simulink model "cruise_control"  (Simulink 7.8)
settings: Solver=FixedStepDiscrete  SolverMode=SingleTasking  StartTime=0.0  StopTime=50  FixedStep=0.01  RelTol=1e-3  AbsTol=1e-6
model workspace (MAT data in the model file):
  converter_data = [0  137.465208994  2.232; 0.1  137.065019157  2.075; 0.2  135.864449646  1.975; 0.3  135.664354728  1.846; 0.4  137.565256453  1.72; 0.5  140.366585312  1.564; 0.6  145.268910814  1.409; 0.7  152.872517717  1.254; 0.8  162.9773111  1.096; 0.81  164.27792807  1.08; 0.82  166.178829795  1.061; 0.83  167.979684062  1.043; 0.84  170.080680706  1.028; 0.85  172.781962105  1.012; 0.86  175.383196045  1.002; 0.87  179.585189333  1.002; 0.88  183.587087703  1.001; 0.89  189.890077635  0.998; 0.9  197.693779455  0.999; 0.92  215.902417037  1.001; 0.94  244.515990379  1.002]
  emap = [-40  -44  -49  -53  -57  -61  -65  -70  -74  -78  -82; 215  117  85  66  44  29  10  -2  -13  -22  -32; 245  208  178  148  122  104  85  66  48  33  18; 264  260  241  219  193  167  152  133  119  96  85; 264  279  282  275  260  238  223  208  189  171  152; 267  290  293  297  290  275  260  256  234  212  193; 267  297  305  305  305  301  293  282  267  249  226; 267  301  308  312  319  323  319  316  297  279  253; 267  301  312  319  327  327  327  327  312  293  267; 267  301  312  319  327  334  334  334  319  305  275]
  Iei = 0.0219914882836
  nevec = [800 1200 1600 2000 2400 2800 3200 3600 4000 4400 4800]
  p0 = 0.07934
  p1 = 0.07934
  thvec = [0; 20; 30; 40; 50; 60; 70; 80; 90; 100]
  vehicledata : num (value not decoded)
values from neighbouring files (symbols this model uses):
  cruise_ki = 0.01    [cruise_control_data.m]    (also in fxpdata_simulinkpackage.mat)
  cruise_kp = 0.02    [cruise_control_data.m]    (also in fxpdata_simulinkpackage.mat)
  target_max = 100    [cruise_control_data.m]    (also in fxpdata_simulinkpackage.mat)
  target_min = 30    [cruise_control_data.m]    (also in fxpdata_simulinkpackage.mat)
  throt_max = 100    [cruise_control_data.m]    (also in fxpdata_simulinkpackage.mat)
  throt_min = 0    [cruise_control_data.m]    (also in fxpdata_simulinkpackage.mat)
  vel_dec = 1    [cruise_control_data.m]    (also in fxpdata_simulinkpackage.mat)
  vel_inc = 1    [cruise_control_data.m]    (also in fxpdata_simulinkpackage.mat)
undefined symbols (not defined in the file or in its folder): DiscIntNeverNeededParam
libraries: simulink x1
Description:
  | ƒNƒ‹?[ƒYƒRƒ“ƒgƒ??[ƒ‹ƒ‚ƒfƒ‹
settings Model: MinMaxOverflowLogging=MinMaxAndOverflow  Creator=The MathWorks Inc.  LastModifiedBy=itoy  CovSaveName=covdata_cc  CovMetricSettings=dcmtr  CovHTMLOptions=-aTS=1 -bRG=1 -bTC=1 -hTR=0 -nFC=0 -scm=1 -bcm=1 -xEv=0  ExtModeTrigMode=oneshot  ExtModeArmWhenConnect=off  ExtModeAutoUpdateStatusClock=off
settings DataIOCC: LimitDataPoints=off  SaveFormat=StructureWithTime  SaveOutput=off  SignalLogging=off  DSMLogging=off  SaveTime=off  SignalLoggingName=mysig
settings OptimizationCC: InlineParams=on  UseIntDivNetSlope=on  InlineInvariantSignals=on  EnhancedBackFolding=on  EfficientFloat2IntCast=on  OptimizeModelRefInitCode=on  LifeSpan=1
settings DebuggingCC: SignalInfNanChecking=error  SaveWithParameterizedLinksMsg=none  CheckExecutionContextPreStartOutputMsg=on  CheckExecutionContextRuntimeOutputMsg=on  SolverPrmCheckMsg=none  SingleTaskRateTransMsg=error  IntegerOverflowMsg=error  UniqueDataStoreMsg=error  BusObjectLabelMismatch=error  RootOutportRequireBusObject=error  AssertControl=DisableAll  StrictBusMsg=ErrorOnBusTreatedAsVector  BusNameAdapt=ErrorWithoutRepair  NonBusSignalsTreatedAsBus=error  LoggingUnavailableSignals=none
settings HardwareCC: ProdIntDivRoundTo=Zero  ProdEndianess=LittleEndian  ProdHWDeviceType=NEC->V850  TargetIntDivRoundTo=Zero  TargetEndianess=LittleEndian  TargetHWDeviceType=MATLAB Host
settings ModelReferenceCC: ModelReferenceNumInstancesAllowed=Single
settings SFSimCC: SFSimEcho=off  SimParseCustomCode=off
settings RTWCC: SystemTargetFile=ert.tlc  TemplateMakefile=ert_default_tmf  Description=Real-Time Workshop Embedded Coder  GenerateReport=on  ProcessScript=ert_make_rtw_hook  IncludeHyperlinkInReport=on  LaunchReport=on  IncludeERTFirstTime=on  RTWCompilerOptimization=On
settings CodeAppCC: IgnoreCustomStorageClasses=off
settings ERTTargetCC: MultiwordLength=2048  GenerateSampleERTMain=on  GenerateErtSFunction=on  CreateSILPILBlock=SIL  InlinedParameterPlacement=NonHierarchical  ERTCustomFileTemplate=example_file_process.tlc  ConvertIfToSwitch=off  SuppressUnreachableDefaultCases=off
settings ConfigComp: Description=Design Verifier Custom Configuration Component  DVMaxProcessTime=3000  DVDisplayUnsatisfiableObjectives=on  DVModelCoverageObjectives=MCDC  DVMaxTestCaseSteps=500  DVTestSuiteOptimization=CombinedObjectives  DVSaveReport=on

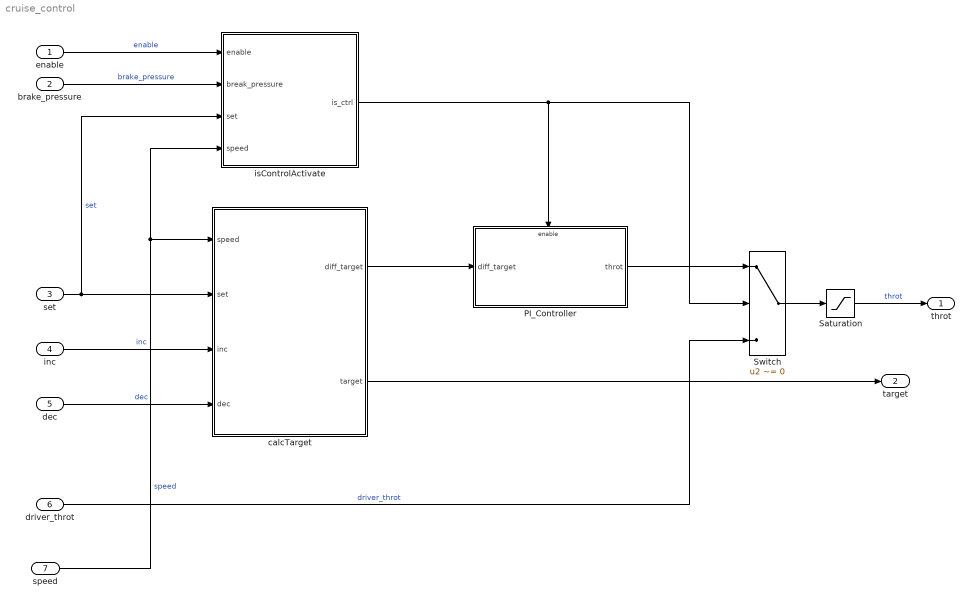
== system cruise_control ==
  enable : Inport  PortDimensions=1  Interpolate=off
  brake_pressure : Inport  Port=2  PortDimensions=1  Interpolate=off
  set : Inport  Port=3  PortDimensions=1  Interpolate=off
  inc : Inport  Port=4  PortDimensions=1  Interpolate=off
  dec : Inport  Port=5  PortDimensions=1  Interpolate=off
  driver_throt : Inport  Port=6  PortDimensions=1  Interpolate=off
  speed : Inport  Port=7  PortDimensions=1  Interpolate=off
  PI_Controller : Subsystem  RequirementInfo={'other' 'cruisecontrol_spec.xls' '@Simulink_requirement_item_13' 'true' 'ƒXƒ?ƒbƒgƒ‹ŒvŽZ' '' ; 'other' 'cruisecontrol_spec.xls' '@Simulink_requirement_item_14' 'true' 'ƒXƒ?ƒbƒgƒ‹’l‚Í?API?§Œä‚É‚æ‚èŒvŽZ‚³‚ê‚é?B' '' } %GIDa_c9cd3625_12f4_4b7c_a41d_1cb041b9c58f
  Saturation : Saturate  RequirementInfo={'other' 'cruisecontrol_spec.xls' '@Simulink_requirement_item_15' 'true' '?o—ÍƒXƒ?ƒbƒgƒ‹’l‚Í?Å‘åƒXƒ?ƒbƒgƒ‹’lˆÈ‰º?A?Å?¬ƒXƒ?ƒbƒgƒ‹’lˆÈ?ã‚Å‚ ‚é?B' '' } %GIDa_29e6bb04_5d3c_40ee_9701_e63e8e51ec96  UpperLimit=throt_max  LowerLimit=throt_min  OutDataTypeStr=Inherit: Inherit via back propagation
      settings: AttributesFormatString=<UpperLimit = %<UpperLimit>>\n<LowerLimit = %<LowerLimit>>
  Switch : Switch  RequirementInfo={'other' 'cruisecontrol_spec.xls' '@Simulink_requirement_item_16' 'true' '?§Œä‹–‰Â‚ªOFF‚Ì?Û‚É‚Í?Aƒhƒ‰ƒCƒo?[ƒXƒ?ƒbƒgƒ‹’l‚ªƒXƒ?ƒbƒgƒ‹’l‚Æ‚µ‚Ä?o—Í‚³‚ê‚é?B' '' } %GIDa_0f4dbb7e_1328_499c_8665_60d1af7bcbda  Criteria=u2 ~= 0  OutDataTypeStr=Inherit: Inherit via back propagation
      settings: AttributesFormatString=<Criteria=%<Criteria>>
  calcTarget : Subsystem  RequirementInfo={'other' 'cruisecontrol_spec.xls' '@Simulink_requirement_item_4' 'true' '–Ú•WŽÔ‘¬?Ý’è' '' } %GIDa_af1ad8a6_b9b3_46e5_9fb4_ba2528b86dbf
  isControlActivate : Subsystem  RequirementInfo={'other' 'cruisecontrol_spec.xls' '@Simulink_requirement_item_1' 'true' 'ƒNƒ‹?[ƒYƒRƒ“ƒgƒ??[ƒ‹—LŒø‰»”»’f' '' ; 'other' 'cruisecontrol_spec.xls' '@Simulink_requirement_item_2' 'true' '?§Œä‹–‰Â‚ÍŽŸ‚Ì?ðŒ?‚ª‘S‚Ä–ž‚½‚³‚ê‚é?ê?‡‚ÉON‚Æ‚È‚é?B ?E—LŒøƒXƒCƒbƒ`‚ªON ?EƒuƒŒ?[ƒL‚ªOFF ?EƒZƒbƒgƒXƒCƒbƒ`‚ªON‚à‚µ‚­‚Í?§Œä‹–‰Â‚Ì‘O‰ñ’l‚ªON ?EŽÔ‘¬‚ª–Ú•W?Å‘åˆÈ‰º‚©‚Â?Å?¬‘¬“xˆÈ?ã' '' } %GIDa_6e4da717_7ca2_4bfc_aa3f_b9dd3e2745f3
  throt : Outport  PortDimensions=[1 1]
  target : Outport  Port=2  PortDimensions=[1 1]
  wires:
  isControlActivate/1(is_ctrl) -> Switch/2, PI_Controller/Enable
  calcTarget/2(target) -> target/1
  calcTarget/1(diff_target) -> PI_Controller/1(diff_target)
  dec/1 -> calcTarget/4(dec)  "dec"
  speed/1 -> isControlActivate/4(speed), calcTarget/1(speed)  "speed"
  inc/1 -> calcTarget/3(inc)  "inc"
  set/1 -> isControlActivate/3(set), calcTarget/2(set)  "set"
  Switch/1 -> Saturation/1
  driver_throt/1 -> Switch/3  "driver_throt"
  brake_pressure/1 -> isControlActivate/2(break_pressure)  "brake_pressure"
  enable/1 -> isControlActivate/1(enable)  "enable"
  PI_Controller/1(throt) -> Switch/1
  Saturation/1 -> throt/1  "throt"

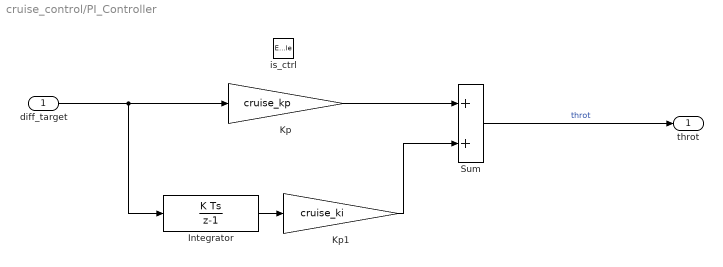
== system cruise_control/PI_Controller ==
  diff_target : Inport
  is_ctrl : EnablePort  StatesWhenEnabling=reset
  Integrator : DiscreteIntegrator  RequirementInfo={'other' 'cruisecontrol_spec.xls' '@Simulink_requirement_item_18' 'true' 'ƒXƒ?ƒbƒgƒ‹’l‚Í?API?§Œä‚É‚æ‚èŒvŽZ‚³‚ê‚é?B' '' } %GIDa_1c8578d3_6938_40c9_979a_c3e32fe3eb66  gainval=1  InitialConditionMode=State only (most efficient)  SampleTime=-1  UpperSaturationLimit=5  LowerSaturationLimit=-5  ICPrevOutput=DiscIntNeverNeededParam  ICPrevScaledInput=DiscIntNeverNeededParam
      settings: AttributesFormatString=<Gain = %<gainval>>\n<%<InitialConditionMode>>\n<SampleTime = %<SampleTime>>
  Kp : Gain  RequirementInfo={'other' 'cruisecontrol_spec.xls' '@Simulink_requirement_item_18' 'true' 'ƒXƒ?ƒbƒgƒ‹’l‚Í?API?§Œä‚É‚æ‚èŒvŽZ‚³‚ê‚é?B' '' } %GIDa_5723d013_10d4_4677_86e7_4397d568c394  Gain=cruise_kp  ParamDataTypeStr=Inherit: Inherit from 'Gain'  OutDataTypeStr=Inherit: Inherit via back propagation
  Kp1 : Gain  RequirementInfo={'other' 'cruisecontrol_spec.xls' '@Simulink_requirement_item_18' 'true' 'ƒXƒ?ƒbƒgƒ‹’l‚Í?API?§Œä‚É‚æ‚èŒvŽZ‚³‚ê‚é?B' '' } %GIDa_289d21ac_7ee3_4a78_ae73_ca0bb78f1562  Gain=cruise_ki  ParamDataTypeStr=Inherit: Inherit from 'Gain'  OutDataTypeStr=Inherit: Inherit via back propagation
  Sum : Sum  RequirementInfo={'other' 'cruisecontrol_spec.xls' '@Simulink_requirement_item_18' 'true' 'ƒXƒ?ƒbƒgƒ‹’l‚Í?API?§Œä‚É‚æ‚èŒvŽZ‚³‚ê‚é?B' '' } %GIDa_d0a7583e_41f1_4826_b25f_6e820e68d741  OutDataTypeStr=Inherit: Inherit via back propagation
  throt : Outport  InitialOutput=0
  wires:
  Kp1/1 -> Sum/2
  Kp/1 -> Sum/1
  Integrator/1 -> Kp1/1
  diff_target/1 -> Kp/1, Integrator/1
  Sum/1 -> throt/1  "throt"

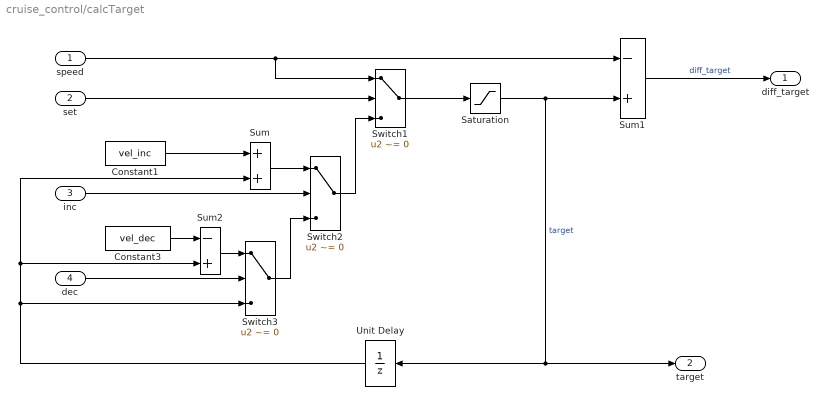
== system cruise_control/calcTarget ==
  speed : Inport
  set : Inport  Port=2
  inc : Inport  Port=3
  dec : Inport  Port=4
  Constant1 : Constant  RequirementInfo={'other' 'cruisecontrol_spec.xls' '@Simulink_requirement_item_9' 'true' '‰Á‘¬ƒXƒCƒbƒ`‚ªON‚Ì?ê?‡‚É‚Í–Ú•WŽÔ‘¬‚Í‘O‰ñ’l‚É‘Î‚µ‚Ä?u‰Á‘¬’l?v‚¾‚¯‘?‰Á‚·‚é?B [?ðŒ?] ?E–Ú•WŽÔ‘¬‚Í?Å‘å‚æ‚è?¬‚©‚Â?Å?¬‚æ‚è‘å ?EƒZƒbƒgƒXƒCƒbƒ`‚ÍOFF' '' } %GIDa_02a51dd8_f8fb_4b58_b24c_edce6b3922af  Value=vel_inc  OutDataTypeStr=Inherit: Inherit via back propagation
  Constant3 : Constant  RequirementInfo={'other' 'cruisecontrol_spec.xls' '@Simulink_requirement_item_8' 'true' 'Œ¸‘¬ƒXƒCƒbƒ`‚ªON‚Ì?ê?‡‚É‚Í–Ú•WŽÔ‘¬‚Í‘O‰ñ’l‚É‘Î‚µ‚Ä?uŒ¸‘¬’l?v‚¾‚¯Œ¸?­‚·‚é?B [?ðŒ?] ?E–Ú•WŽÔ‘¬‚Í?Å‘å‚æ‚è?¬‚©‚Â?Å?¬‚æ‚è‘å ?EƒZƒbƒgƒXƒCƒbƒ`‚ÍOFF' '' } %GIDa_18e49c28_c92c_4a8f_854f_3eb142b3e640  Value=vel_dec  OutDataTypeStr=Inherit: Inherit via back propagation
  Saturation : Saturate  UpperLimit=target_max  LowerLimit=target_min
      settings: AttributesFormatString=<UpperLimit = %<UpperLimit>>\n<LowerLimit = %<LowerLimit>>
  Sum : Sum  RequirementInfo={'other' 'cruisecontrol_spec.xls' '@Simulink_requirement_item_7' 'true' '‰Á‘¬ƒXƒCƒbƒ`‚ªON‚Ì?ê?‡‚É‚Í–Ú•WŽÔ‘¬‚Í‘O‰ñ’l‚É‘Î‚µ‚Ä?u‰Á‘¬’l?v‚¾‚¯‘?‰Á‚·‚é?B [?ðŒ?] ?E–Ú•WŽÔ‘¬‚Í?Å‘å‚æ‚è?¬‚©‚Â?Å?¬‚æ‚è‘å ?EƒZƒbƒgƒXƒCƒbƒ`‚ÍOFF' '' } %GIDa_944f99be_7e99_4675_b148_a5aefe76214d
  Sum1 : Sum  RequirementInfo={'other' 'cruisecontrol_spec.xls' '@Simulink_requirement_item_12' 'true' '–Ú•WŽÔ‘¬?·‚Í?A–Ú•WŽÔ‘¬ - ŽÔ‘¬‚Å‚ ‚é?B [‘O’ñ?ðŒ?] ?E–Ú•WŽÔ‘¬‚Í?Å‘å‚æ‚è?¬‚©‚Â?Å?¬‚æ‚è‘å' '' } %GIDa_e986365a_a7ea_41b2_bba3_c777d3b062b4  Inputs=-+  OutDataTypeStr=Inherit: Same as first input
  Sum2 : Sum  RequirementInfo={'other' 'cruisecontrol_spec.xls' '@Simulink_requirement_item_8' 'true' 'Œ¸‘¬ƒXƒCƒbƒ`‚ªON‚Ì?ê?‡‚É‚Í–Ú•WŽÔ‘¬‚Í‘O‰ñ’l‚É‘Î‚µ‚Ä?uŒ¸‘¬’l?v‚¾‚¯Œ¸?­‚·‚é?B [?ðŒ?] ?E–Ú•WŽÔ‘¬‚Í?Å‘å‚æ‚è?¬‚©‚Â?Å?¬‚æ‚è‘å ?EƒZƒbƒgƒXƒCƒbƒ`‚ÍOFF' '' } %GIDa_0cb061b8_d2f3_4670_9f86_c1320ad3b822  Inputs=-+
  Switch1 : Switch  RequirementInfo={'other' 'cruisecontrol_spec.xls' '@Simulink_requirement_item_5' 'true' 'ƒZƒbƒgƒXƒCƒbƒ`‚ªON‚Ì?ê?‡‚É‚Í–Ú•WŽÔ‘¬‚ÍŒ»?Ý‚ÌŽÔ‘¬‚Æ‚È‚é [?ðŒ?] ?E–Ú•WŽÔ‘¬‚Í?Å‘å‚æ‚è?¬‚©‚Â?Å?¬‚æ‚è‘å' '' } %GIDa_1ae4a051_4e80_4bd0_935d_80110ada8620  Criteria=u2 ~= 0
      settings: AttributesFormatString=<Criteria=%<Criteria>>
  Switch2 : Switch  RequirementInfo={'other' 'cruisecontrol_spec.xls' '@Simulink_requirement_item_6' 'true' 'ƒZƒbƒgƒXƒCƒbƒ`‚Í‰Á‘¬ƒXƒCƒbƒ`‚¨‚æ‚ÑŒ¸‘¬ƒXƒCƒbƒ`‚æ‚è—D?æ‚³‚ê‚é' '' ; 'other' 'cruisecontrol_spec.xls' '@Simulink_requirement_item_7' 'true' '‰Á‘¬ƒXƒCƒbƒ`‚ªON‚Ì?ê?‡‚É‚Í–Ú•WŽÔ‘¬‚Í‘O‰ñ’l‚É‘Î‚µ‚Ä?u‰Á‘¬’l?v‚¾‚¯‘?‰Á‚·‚é?B [?ðŒ?] ?E–Ú•WŽÔ‘¬‚Í?Å‘å‚æ‚è?¬‚©‚Â?Å?¬‚æ‚è‘å ?EƒZƒbƒgƒXƒCƒbƒ`‚ÍOFF' '' ; 'other' 'cruisecontrol_spec.xls' '@Simulink_requirement_item_10' 'true' '‰Á‘¬ƒXƒCƒbƒ`‚ÍŒ¸‘¬ƒXƒCƒbƒ`‚æ‚è—D?æ‚³‚ê‚é' '' } %GIDa_acacb1c5_12a2_4ae3_823a_d0515386cbda  Criteria=u2 ~= 0
      settings: AttributesFormatString=<Criteria=%<Criteria>>
  Switch3 : Switch  RequirementInfo={'other' 'cruisecontrol_spec.xls' '@Simulink_requirement_item_6' 'true' 'ƒZƒbƒgƒXƒCƒbƒ`‚Í‰Á‘¬ƒXƒCƒbƒ`‚¨‚æ‚ÑŒ¸‘¬ƒXƒCƒbƒ`‚æ‚è—D?æ‚³‚ê‚é' '' ; 'other' 'cruisecontrol_spec.xls' '@Simulink_requirement_item_8' 'true' 'Œ¸‘¬ƒXƒCƒbƒ`‚ªON‚Ì?ê?‡‚É‚Í–Ú•WŽÔ‘¬‚Í‘O‰ñ’l‚É‘Î‚µ‚Ä?uŒ¸‘¬’l?v‚¾‚¯Œ¸?­‚·‚é?B [?ðŒ?] ?E–Ú•WŽÔ‘¬‚Í?Å‘å‚æ‚è?¬‚©‚Â?Å?¬‚æ‚è‘å ?EƒZƒbƒgƒXƒCƒbƒ`‚ÍOFF' '' ; 'other' 'cruisecontrol_spec.xls' '@Simulink_requirement_item_10' 'true' '‰Á‘¬ƒXƒCƒbƒ`‚ÍŒ¸‘¬ƒXƒCƒbƒ`‚æ‚è—D?æ‚³‚ê‚é' '' ; 'other' 'cruisecontrol_spec.xls' '@Simulink_requirement_item_11' 'true' '‰Á‘¬ƒXƒCƒbƒ`‚¨‚æ‚ÑŒ¸‘¬ƒXƒCƒbƒ`‚ª‹¤‚É–³Œø‚Ì?ê?‡?A–Ú•WŽÔ‘¬‚Í‘O‰ñ’l‚ð—p‚¢‚é [‘O’ñ?ðŒ?] ?EƒZƒbƒgƒXƒCƒbƒ`‚ÍOFF ?E–Ú•WŽÔ‘¬‚Í?Å‘å‚æ‚è?¬‚©‚Â?Å?¬‚æ‚è‘å' '' } %GIDa_9787d40d_5041_4fab_8b80_2982d0f9111f  Criteria=u2 ~= 0
      settings: AttributesFormatString=<Criteria=%<Criteria>>
  Unit Delay : UnitDelay  SampleTime=-1
  diff_target : Outport
  target : Outport  Port=2
  wires:
  Saturation/1 -> Sum1/2, target/1, Unit Delay/1  "target"
  set/1 -> Switch1/2
  speed/1 -> Switch1/1, Sum1/1
  inc/1 -> Switch2/2
  Constant1/1 -> Sum/1
  Sum/1 -> Switch2/1
  dec/1 -> Switch3/2
  Constant3/1 -> Sum2/1
  Sum2/1 -> Switch3/1
  Switch2/1 -> Switch1/3
  Switch3/1 -> Switch2/3
  Unit Delay/1 -> Switch3/3, Sum2/2, Sum/2
  Switch1/1 -> Saturation/1
  Sum1/1 -> diff_target/1  "diff_target"

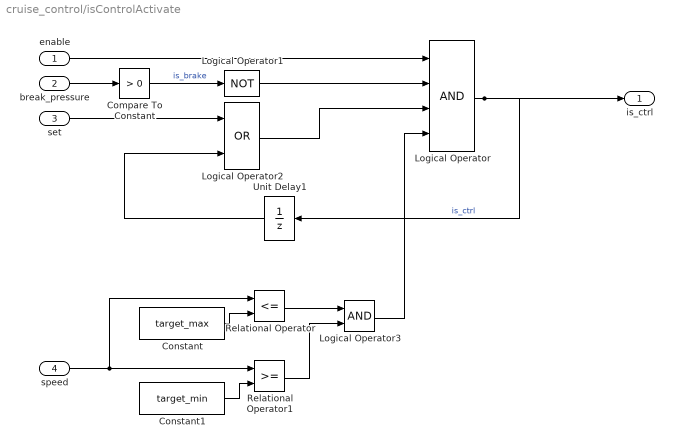
== system cruise_control/isControlActivate ==
  enable : Inport
  break_pressure : Inport  Port=2
  set : Inport  Port=3
  speed : Inport  Port=4
  Compare To Constant : simulink/Logic and Bit Operations/Compare To Constant  RequirementInfo={'other' 'cruisecontrol_spec.xls' '@Simulink_requirement_item_17' 'true' '?§Œä‹–‰Â‚ÍŽŸ‚Ì?ðŒ?‚ª‘S‚Ä–ž‚½‚³‚ê‚é?ê?‡‚ÉON‚Æ‚È‚é?B ?E—LŒøƒXƒCƒbƒ`‚ªON ?EƒuƒŒ?[ƒL‚ªOFF ?EƒZƒbƒgƒXƒCƒbƒ`‚ªON‚à‚µ‚­‚Í?§Œä‹–‰Â‚Ì‘O‰ñ’l‚ªON ?EŽÔ‘¬‚ª–Ú•W?Å‘åˆÈ‰º‚©‚Â?Å?¬‘¬“xˆÈ?ã' '' } %GIDa_e732d17b_1fa4_4dc8_8756_ac241ba75088  relop=>  const=0  OutDataTypeStr=uint8
  Constant : Constant  RequirementInfo={'other' 'cruisecontrol_spec.xls' '@Simulink_requirement_item_17' 'true' '?§Œä‹–‰Â‚ÍŽŸ‚Ì?ðŒ?‚ª‘S‚Ä–ž‚½‚³‚ê‚é?ê?‡‚ÉON‚Æ‚È‚é?B ?E—LŒøƒXƒCƒbƒ`‚ªON ?EƒuƒŒ?[ƒL‚ªOFF ?EƒZƒbƒgƒXƒCƒbƒ`‚ªON‚à‚µ‚­‚Í?§Œä‹–‰Â‚Ì‘O‰ñ’l‚ªON ?EŽÔ‘¬‚ª–Ú•W?Å‘åˆÈ‰º‚©‚Â?Å?¬‘¬“xˆÈ?ã' '' } %GIDa_5046f154_2f2e_4946_843e_e38a88e06dd9  Value=target_max
  Constant1 : Constant  RequirementInfo={'other' 'cruisecontrol_spec.xls' '@Simulink_requirement_item_17' 'true' '?§Œä‹–‰Â‚ÍŽŸ‚Ì?ðŒ?‚ª‘S‚Ä–ž‚½‚³‚ê‚é?ê?‡‚ÉON‚Æ‚È‚é?B ?E—LŒøƒXƒCƒbƒ`‚ªON ?EƒuƒŒ?[ƒL‚ªOFF ?EƒZƒbƒgƒXƒCƒbƒ`‚ªON‚à‚µ‚­‚Í?§Œä‹–‰Â‚Ì‘O‰ñ’l‚ªON ?EŽÔ‘¬‚ª–Ú•W?Å‘åˆÈ‰º‚©‚Â?Å?¬‘¬“xˆÈ?ã' '' } %GIDa_776ebf55_8cd9_493d_ac8e_7f437ae053fb  Value=target_min
  Logical Operator : Logic  RequirementInfo={'other' 'cruisecontrol_spec.xls' '@Simulink_requirement_item_17' 'true' '?§Œä‹–‰Â‚ÍŽŸ‚Ì?ðŒ?‚ª‘S‚Ä–ž‚½‚³‚ê‚é?ê?‡‚ÉON‚Æ‚È‚é?B ?E—LŒøƒXƒCƒbƒ`‚ªON ?EƒuƒŒ?[ƒL‚ªOFF ?EƒZƒbƒgƒXƒCƒbƒ`‚ªON‚à‚µ‚­‚Í?§Œä‹–‰Â‚Ì‘O‰ñ’l‚ªON ?EŽÔ‘¬‚ª–Ú•W?Å‘åˆÈ‰º‚©‚Â?Å?¬‘¬“xˆÈ?ã' '' } %GIDa_f3c59dc0_ed0b_409b_9647_e5f2140a460b  Inputs=4  AllPortsSameDT=off  OutDataTypeStr=boolean
  Logical Operator1 : Logic  RequirementInfo={'other' 'cruisecontrol_spec.xls' '@Simulink_requirement_item_17' 'true' '?§Œä‹–‰Â‚ÍŽŸ‚Ì?ðŒ?‚ª‘S‚Ä–ž‚½‚³‚ê‚é?ê?‡‚ÉON‚Æ‚È‚é?B ?E—LŒøƒXƒCƒbƒ`‚ªON ?EƒuƒŒ?[ƒL‚ªOFF ?EƒZƒbƒgƒXƒCƒbƒ`‚ªON‚à‚µ‚­‚Í?§Œä‹–‰Â‚Ì‘O‰ñ’l‚ªON ?EŽÔ‘¬‚ª–Ú•W?Å‘åˆÈ‰º‚©‚Â?Å?¬‘¬“xˆÈ?ã' '' } %GIDa_872b54d0_1b90_4f2d_a3a3_599e08d9785c  Operator=NOT  AllPortsSameDT=off  OutDataTypeStr=boolean
  Logical Operator2 : Logic  RequirementInfo={'other' 'cruisecontrol_spec.xls' '@Simulink_requirement_item_17' 'true' '?§Œä‹–‰Â‚ÍŽŸ‚Ì?ðŒ?‚ª‘S‚Ä–ž‚½‚³‚ê‚é?ê?‡‚ÉON‚Æ‚È‚é?B ?E—LŒøƒXƒCƒbƒ`‚ªON ?EƒuƒŒ?[ƒL‚ªOFF ?EƒZƒbƒgƒXƒCƒbƒ`‚ªON‚à‚µ‚­‚Í?§Œä‹–‰Â‚Ì‘O‰ñ’l‚ªON ?EŽÔ‘¬‚ª–Ú•W?Å‘åˆÈ‰º‚©‚Â?Å?¬‘¬“xˆÈ?ã' '' } %GIDa_9aba9474_4942_4c34_9f42_e08d8d74ad04  Operator=OR  AllPortsSameDT=off  OutDataTypeStr=boolean
  Logical Operator3 : Logic  RequirementInfo={'other' 'cruisecontrol_spec.xls' '@Simulink_requirement_item_17' 'true' '?§Œä‹–‰Â‚ÍŽŸ‚Ì?ðŒ?‚ª‘S‚Ä–ž‚½‚³‚ê‚é?ê?‡‚ÉON‚Æ‚È‚é?B ?E—LŒøƒXƒCƒbƒ`‚ªON ?EƒuƒŒ?[ƒL‚ªOFF ?EƒZƒbƒgƒXƒCƒbƒ`‚ªON‚à‚µ‚­‚Í?§Œä‹–‰Â‚Ì‘O‰ñ’l‚ªON ?EŽÔ‘¬‚ª–Ú•W?Å‘åˆÈ‰º‚©‚Â?Å?¬‘¬“xˆÈ?ã' '' } %GIDa_bb979064_f76e_411f_b388_1ad8c0cd6042  AllPortsSameDT=off  OutDataTypeStr=boolean
  Relational Operator : RelationalOperator  RequirementInfo={'other' 'cruisecontrol_spec.xls' '@Simulink_requirement_item_17' 'true' '?§Œä‹–‰Â‚ÍŽŸ‚Ì?ðŒ?‚ª‘S‚Ä–ž‚½‚³‚ê‚é?ê?‡‚ÉON‚Æ‚È‚é?B ?E—LŒøƒXƒCƒbƒ`‚ªON ?EƒuƒŒ?[ƒL‚ªOFF ?EƒZƒbƒgƒXƒCƒbƒ`‚ªON‚à‚µ‚­‚Í?§Œä‹–‰Â‚Ì‘O‰ñ’l‚ªON ?EŽÔ‘¬‚ª–Ú•W?Å‘åˆÈ‰º‚©‚Â?Å?¬‘¬“xˆÈ?ã' '' } %GIDa_a3669dc6_30cc_496e_9921_e3238a4912bb  Operator=<=  OutDataTypeStr=boolean
  Relational Operator1 : RelationalOperator  RequirementInfo={'other' 'cruisecontrol_spec.xls' '@Simulink_requirement_item_17' 'true' '?§Œä‹–‰Â‚ÍŽŸ‚Ì?ðŒ?‚ª‘S‚Ä–ž‚½‚³‚ê‚é?ê?‡‚ÉON‚Æ‚È‚é?B ?E—LŒøƒXƒCƒbƒ`‚ªON ?EƒuƒŒ?[ƒL‚ªOFF ?EƒZƒbƒgƒXƒCƒbƒ`‚ªON‚à‚µ‚­‚Í?§Œä‹–‰Â‚Ì‘O‰ñ’l‚ªON ?EŽÔ‘¬‚ª–Ú•W?Å‘åˆÈ‰º‚©‚Â?Å?¬‘¬“xˆÈ?ã' '' } %GIDa_5d40086f_aa9e_4d24_9f7d_0832032cf57a  OutDataTypeStr=boolean
  Unit Delay1 : UnitDelay  RequirementInfo={'other' 'cruisecontrol_spec.xls' '@Simulink_requirement_item_3' 'true' '?‰Šú?ðŒ?‚Å‚ÍƒZƒbƒgƒXƒCƒbƒ`‚ªON‚Å‚È‚¢ŒÀ‚è?§Œä‹–‰Â‚Í–³Œø‚Å‚ ‚é' '' } %GIDa_df4d3851_f015_45c6_a07c_a3aea4ec8833  SampleTime=-1
  is_ctrl : Outport
  wires:
  Compare To Constant/1 -> Logical Operator1/1  "is_brake"
  Constant/1 -> Relational Operator/2
  Logical Operator3/1 -> Logical Operator/4
  Relational Operator1/1 -> Logical Operator3/2
  Relational Operator/1 -> Logical Operator3/1
  speed/1 -> Relational Operator/1, Relational Operator1/1
  Constant1/1 -> Relational Operator1/2
  break_pressure/1 -> Compare To Constant/1
  enable/1 -> Logical Operator/1
  set/1 -> Logical Operator2/1
  Logical Operator1/1 -> Logical Operator/2
  Logical Operator2/1 -> Logical Operator/3
  Unit Delay1/1 -> Logical Operator2/2
  Logical Operator/1 -> is_ctrl/1, Unit Delay1/1  "is_ctrl"
